simulink model "svm_mstab"  (Simulink 8.6)
settings: Solver=VariableStepAuto  StartTime=0.0  StopTime=10.0  RelTol=1e-3
values from neighbouring files (symbols this model uses):
  M_psderivative = ss(blkdiag(T_psderivative, T_psderivative, T_psderivative))    [svm_buildLinearControllers.m]
  My = ss(tf([eye(6) -eye(6)]))    [svm_buildLinearControllers.m]
  Mz = ss(tf([pickP, -pickP]))    [svm_buildLinearControllers.m]
settings Model: Creator=j.bolting  LastModifiedBy=j.bolting
settings DataIOCC: SaveFormat=Dataset  SignalLoggingSaveFormat=Dataset
settings OptimizationCC: DefaultParameterBehavior=Inlined  BufferReuse=off  ExpressionDepthLimit=128
settings DebuggingCC: UnderspecifiedInitializationDetection=Simplified  MergeDetectMultiDrivingBlocksExec=error  SolverPrmCheckMsg=none  FcnCallInpInsideContextMsg=EnableAllAsError  StateNameClashWarn=none  InitInArrayFormatMsg=none
settings HardwareCC: ProdBitPerPointer=64  ProdLargestAtomicFloat=Float  ProdIntDivRoundTo=Zero  ProdEndianess=LittleEndian  ProdWordSize=64  ProdHWDeviceType=Intel->x86-64 (Windows64)
settings GRTTargetCC: GeneratePreprocessorConditionals=Use local settings  CombineOutputUpdateFcns=on  GRTInterface=off
settings ConfigComp: CovModelRefEnable=off

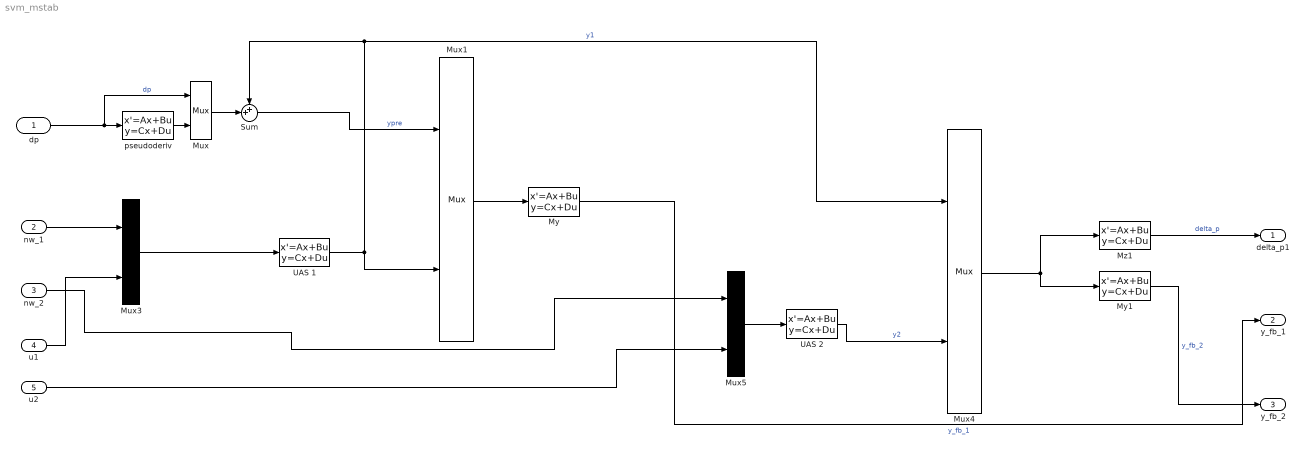
== system svm_mstab ==
  dp : Inport  PortDimensions=2
  nw_1 : Inport  Port=2  PortDimensions=2
  nw_2 : Inport  Port=3  PortDimensions=2
  u1 : Inport  Port=4  PortDimensions=2
  u2 : Inport  Port=5  PortDimensions=2
  Mux{,1,3..5} (5 alike) : Mux  Inputs=2
  My : StateSpace  A=My.a  B=My.b  C=My.c  D=My.d  X0=0
  My1 : StateSpace  A=My.a  B=My.b  C=My.c  D=My.d  X0=0
  Mz1 : StateSpace  A=Mz.a  B=Mz.b  C=Mz.c  D=Mz.d  X0=0
  Sum : Sum  Inputs=++|
  UAS 1 : StateSpace  A=uavsim.svm.linearmodels.sorder_longi.airspeed_15.a  B=uavsim.svm.linearmodels.sorder_longi.airspeed_15.b  C=uavsim.svm.linearmodels.sorder_longi.airspeed_15.c  D=uavsim.svm.linearmodels.sorder_longi.airspeed_15.d  X0=0
  UAS 2 : StateSpace  A=uavsim.svm.linearmodels.sorder_longi.airspeed_15.a  B=uavsim.svm.linearmodels.sorder_longi.airspeed_15.b  C=uavsim.svm.linearmodels.sorder_longi.airspeed_15.c  D=uavsim.svm.linearmodels.sorder_longi.airspeed_15.d  X0=0
  pseudoderiv : StateSpace  A=M_psderivative.a  B=M_psderivative.b  C=M_psderivative.c  D=M_psderivative.d  X0=0
  delta_p1 : Outport
  y_fb_1 : Outport  Port=2
  y_fb_2 : Outport  Port=3
  wires:
  dp/1 -> pseudoderiv/1, Mux/1  "dp"
  pseudoderiv/1 -> Mux/2
  Mux/1 -> Sum/2
  nw_1/1 -> Mux3/1
  u1/1 -> Mux3/2
  Mux3/1 -> UAS 1/1
  Sum/1 -> Mux1/1  "ypre"
  Mux1/1 -> My/1
  My/1 -> y_fb_1/1  "y_fb_1"
  nw_2/1 -> Mux5/1
  u2/1 -> Mux5/2
  Mux5/1 -> UAS 2/1
  UAS 1/1 -> Mux4/1, Sum/1, Mux1/2  "y1"
  UAS 2/1 -> Mux4/2  "y2"
  Mux4/1 -> Mz1/1, My1/1
  Mz1/1 -> delta_p1/1  "delta_p"
  My1/1 -> y_fb_2/1  "y_fb_2"
